simulink library "helperLib"  (R2016a)
settings: Solver=ode45  StartTime=0.0  StopTime=10.0  RelTol=1e-3
values from neighbouring files (symbols this model uses):
  atanDomain = 5    [rev0BB_setup.m]
  atanResolution = 2^-9    (= 0.001953125)    [rev0BB_setup.m]
  averaging_denom = zeros(1, averaging_samples)    [rev0BB_setup.m]
  averaging_num = ones(1, averaging_samples)    [rev0BB_setup.m]
  frac_lut_domain = 256    [rev0BB_setup.m]
  frac_lut_res = 2^-5    (= 0.03125)    [rev0BB_setup.m]
  mult_pipeline = 1    [rev0BB_setup.m]
  regular_pipeline = 1    [rev0BB_setup.m]
libraries: helperLib x11, simulink x8
settings Model: Creator=cyarp  LastModifiedBy=Christopher Yarp
settings DataIOCC: LimitDataPoints=on  SaveFormat=Array
settings DebuggingCC: SolverPrmCheckMsg=warning
settings HardwareCC: ProdBitPerPointer=32  ProdLargestAtomicFloat=None  ProdIntDivRoundTo=Undefined  ProdEndianess=Unspecified  ProdWordSize=32  ProdHWDeviceType=32-bit Generic
settings ModelReferenceCC: PropagateSignalLabelsOutOfModel=off
settings ConfigComp: CovModelRefEnable=Off  CovSFcnEnable=off

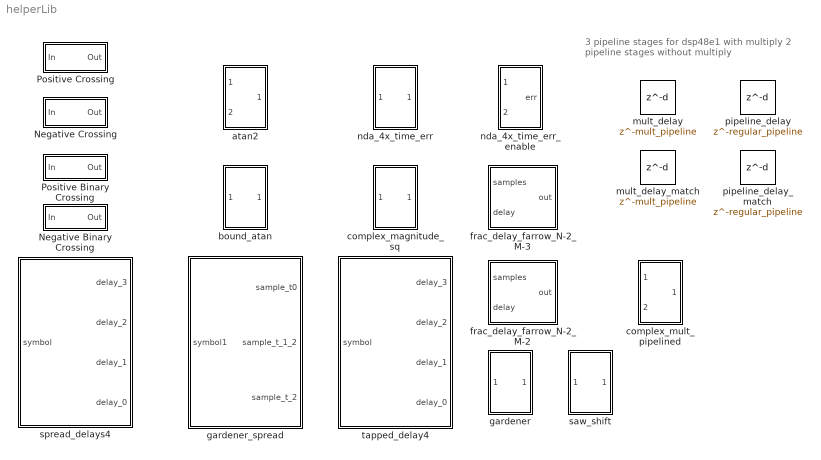
== system helperLib ==
  note: 3 pipeline stages for dsp48e1 with multiply
      | 2 pipeline stages without multiply
  Negative Binary Crossing : Subsystem
  Negative Crossing : Subsystem  mask{crossPt=0}
      mask prompts: crossPt "Crossing Point"
      mask help:
      | Negative Crossing
      | Will output true if goes greater than or equal to threshold to less than
      | theshold.  Will output zero otherwise.
      mask Display: fprintf('-Cross (%d)', crossPt)
  Positive Binary Crossing : Subsystem
  Positive Crossing : Subsystem  mask{crossPt=0}
      mask prompts: crossPt "Crossing Pt"
      mask help:
      | Positive Crossing
      | Will output true if goes from below threshold to greater than or equal to
      | theshold.  Will output zero otherwise.
      mask Display: fprintf('+Cross (%d)', crossPt)
  atan2 : Subsystem
  bound_atan : Subsystem
  complex_magnitude_sq : Subsystem
  complex_mult_pipelined : Subsystem
  frac_delay_farrow_N-2_M-2 : Subsystem
  frac_delay_farrow_N-2_M-3 : Subsystem
  gardener : Subsystem
  gardener_spread : Subsystem
  mult_delay : Delay  DelayLength=mult_pipeline
  mult_delay_match : Delay  DelayLength=mult_pipeline
  nda_4x_time_err : Subsystem
  nda_4x_time_err_enable : Subsystem
  pipeline_delay : Delay  DelayLength=regular_pipeline
  pipeline_delay_match : Delay  DelayLength=regular_pipeline
  saw_shift : Subsystem
  spread_delays4 : Subsystem
  "tapped_delay4 " : Subsystem

== system helperLib/Negative Binary Crossing ==
  In : Inport  OutDataTypeStr=boolean
  Delay : Delay  DelayLength=1  InitialCondition=0
  Logical Operator : Logic  AllPortsSameDT=off  OutDataTypeStr=boolean
  Logical Operator1 : Logic  Operator=NOT  Inputs=1  AllPortsSameDT=off  OutDataTypeStr=boolean
  Out : Outport  OutDataTypeStr=boolean
  wires:
  In/1 -> Logical Operator1/1, Delay/1
  Logical Operator/1 -> Out/1
  Logical Operator1/1 -> Logical Operator/1
  Delay/1 -> Logical Operator/2

== system helperLib/Negative Crossing ==
  In : Inport
  Compare To Constant : simulink/Logic and Bit Operations/Compare To Constant  relop=<  const=crossPt  OutDataTypeStr=boolean
  Compare To Constant1 : simulink/Logic and Bit Operations/Compare To Constant  relop=>=  const=crossPt  OutDataTypeStr=boolean
  Delay : Delay  DelayLength=1  InitialCondition=0
  Logical Operator : Logic  AllPortsSameDT=off  OutDataTypeStr=boolean
  Out : Outport  OutDataTypeStr=boolean
  wires:
  Logical Operator/1 -> Out/1
  In/1 -> Compare To Constant1/1, Compare To Constant/1
  Compare To Constant/1 -> Logical Operator/1
  Compare To Constant1/1 -> Delay/1
  Delay/1 -> Logical Operator/2

== system helperLib/Positive Binary Crossing ==
  In : Inport  OutDataTypeStr=boolean
  Delay : Delay  DelayLength=1  InitialCondition=0
  Logical Operator : Logic  AllPortsSameDT=off  OutDataTypeStr=boolean
  Logical Operator1 : Logic  Operator=NOT  Inputs=1  AllPortsSameDT=off  OutDataTypeStr=boolean
  Out : Outport  OutDataTypeStr=boolean
  wires:
  In/1 -> Logical Operator/1, Delay/1
  Logical Operator/1 -> Out/1
  Delay/1 -> Logical Operator1/1
  Logical Operator1/1 -> Logical Operator/2

== system helperLib/Positive Crossing ==
  In : Inport
  Compare To Constant : simulink/Logic and Bit Operations/Compare To Constant  relop=>=  const=crossPt  OutDataTypeStr=boolean
  Compare To Constant1 : simulink/Logic and Bit Operations/Compare To Constant  relop=<  const=crossPt  OutDataTypeStr=boolean
  Delay : Delay  DelayLength=1  InitialCondition=0
  Logical Operator : Logic  AllPortsSameDT=off  OutDataTypeStr=boolean
  Out : Outport  OutDataTypeStr=boolean
  wires:
  Compare To Constant1/1 -> Delay/1
  Compare To Constant/1 -> Logical Operator/1
  Logical Operator/1 -> Out/1
  In/1 -> Compare To Constant1/1, Compare To Constant/1
  Delay/1 -> Logical Operator/2

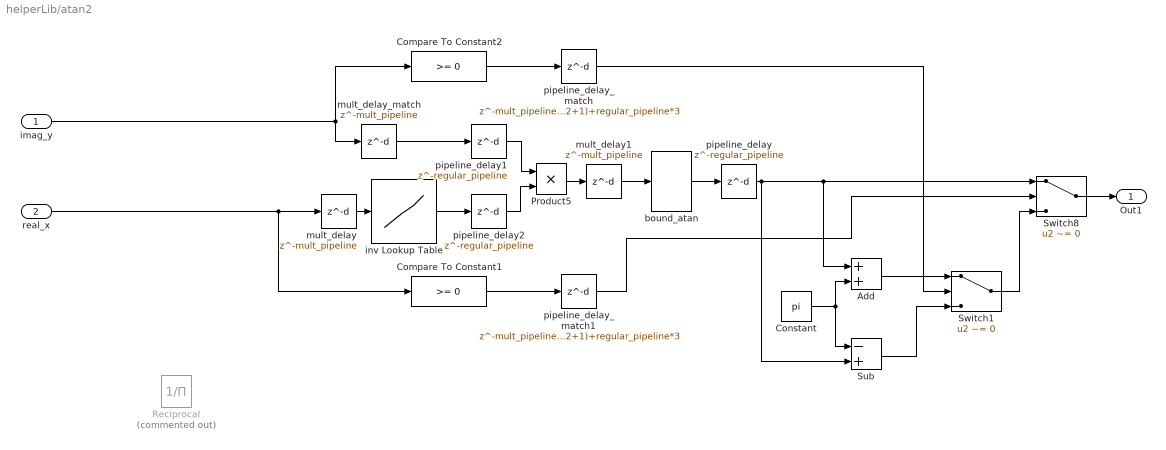
== system helperLib/atan2 ==
  imag_y : Inport
  real_x : Inport  Port=2
  Add : Sum
  Compare To Constant1 : simulink/Logic and Bit Operations/Compare To Constant  relop=>=  const=0  OutDataTypeStr=boolean
  Compare To Constant2 : simulink/Logic and Bit Operations/Compare To Constant  relop=>=  const=0  OutDataTypeStr=boolean
  Constant : Constant  Value=pi  OutDataTypeStr=Inherit: Inherit via back propagation  SampleTime=-1
  Product5 : Product  OutDataTypeStr=Inherit: Same as first input
  Reciprocal : Product  Commented=on  Inputs=/  SaturateOnIntegerOverflow=on  RndMeth=Zero
  Sub : Sum  Inputs=-+
  Switch1 : Switch  Criteria=u2 ~= 0  OutDataTypeStr=Inherit: Inherit via back propagation
  Switch8 : Switch  Criteria=u2 ~= 0  OutDataTypeStr=Inherit: Inherit via back propagation
  bound_atan : helperLib/bound_atan
  inv Lookup Table : Lookup_n-D  NumberOfTableDimensions=1  BreakpointsForDimension1=-frac_lut_domain:frac_lut_res:frac_lut_domain  IndexSearchMethod=Evenly spaced points  Table=ones(size(-frac_lut_domain:frac_lut_res:frac_lut_domain))./(-frac_lut_domain:frac_lut_res:frac_lut_domain)  InterpMethod=Flat  DiagnosticForOutOfRangeInput=Error  InternalRulePriority=Speed  RndMeth=Simplest  InputSameDT=on
  mult_delay : Delay  DelayLength=mult_pipeline
  mult_delay1 : Delay  DelayLength=mult_pipeline
  mult_delay_match : Delay  DelayLength=mult_pipeline
  pipeline_delay : Delay  DelayLength=regular_pipeline
  pipeline_delay1 : Delay  DelayLength=regular_pipeline
  pipeline_delay2 : Delay  DelayLength=regular_pipeline
  pipeline_delay_match : Delay  DelayLength=mult_pipeline*(2+1)+regular_pipeline*3
  pipeline_delay_match1 : Delay  DelayLength=mult_pipeline*(2+1)+regular_pipeline*3
  Out1 : Outport
  wires:
  inv Lookup Table/1 -> pipeline_delay2/1
  Product5/1 -> mult_delay1/1
  bound_atan/1 -> pipeline_delay/1
  mult_delay_match/1 -> pipeline_delay1/1
  pipeline_delay/1 -> Sub/2, Add/1, Switch8/1
  Compare To Constant1/1 -> pipeline_delay_match1/1
  Compare To Constant2/1 -> pipeline_delay_match/1
  Switch1/1 -> Switch8/3
  Add/1 -> Switch1/1
  Constant/1 -> Add/2, Sub/1
  Sub/1 -> Switch1/3
  Switch8/1 -> Out1/1
  imag_y/1 -> mult_delay_match/1, Compare To Constant2/1
  pipeline_delay_match1/1 -> Switch8/2
  pipeline_delay_match/1 -> Switch1/2
  real_x/1 -> mult_delay/1, Compare To Constant1/1
  mult_delay/1 -> inv Lookup Table/1
  pipeline_delay1/1 -> Product5/1
  pipeline_delay2/1 -> Product5/2
  mult_delay1/1 -> bound_atan/1

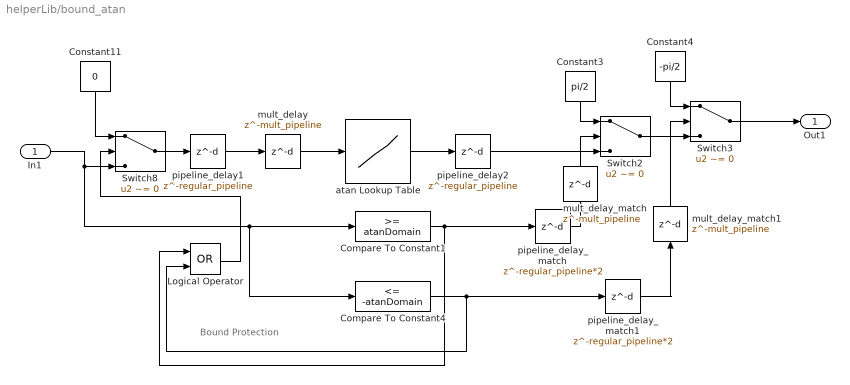
== system helperLib/bound_atan ==
  note: Bound Protection
  In1 : Inport
  Compare To Constant1 : simulink/Logic and Bit Operations/Compare To Constant  relop=>=  const=atanDomain  OutDataTypeStr=boolean
  Compare To Constant4 : simulink/Logic and Bit Operations/Compare To Constant  relop=<=  const=-atanDomain  OutDataTypeStr=boolean
  Constant11 : Constant  Value=0  OutDataTypeStr=Inherit: Inherit via back propagation  SampleTime=-1
  Constant3 : Constant  Value=pi/2  OutDataTypeStr=Inherit: Inherit via back propagation  SampleTime=-1
  Constant4 : Constant  Value=-pi/2  OutDataTypeStr=Inherit: Inherit via back propagation  SampleTime=-1
  Logical Operator : Logic  Operator=OR  AllPortsSameDT=off  OutDataTypeStr=boolean
  Switch2 : Switch  Criteria=u2 ~= 0  OutDataTypeStr=Inherit: Inherit via back propagation
  Switch3 : Switch  Criteria=u2 ~= 0  OutDataTypeStr=Inherit: Inherit via back propagation
  Switch8 : Switch  Criteria=u2 ~= 0  OutDataTypeStr=Inherit: Inherit via back propagation
  atan Lookup Table : Lookup_n-D  NumberOfTableDimensions=1  BreakpointsForDimension1=[-atanDomain:atanResolution:atanDomain]  IndexSearchMethod=Evenly spaced points  Table=atan([-atanDomain:atanResolution:atanDomain])  InterpMethod=Flat  DiagnosticForOutOfRangeInput=Error  RemoveProtectionInput=on  InternalRulePriority=Speed  RndMeth=Simplest  InputSameDT=on
  mult_delay : Delay  DelayLength=mult_pipeline
  mult_delay_match : Delay  DelayLength=mult_pipeline
  mult_delay_match1 : Delay  DelayLength=mult_pipeline
  pipeline_delay1 : Delay  DelayLength=regular_pipeline
  pipeline_delay2 : Delay  DelayLength=regular_pipeline
  pipeline_delay_match : Delay  DelayLength=regular_pipeline*2
  pipeline_delay_match1 : Delay  DelayLength=regular_pipeline*2
  Out1 : Outport
  wires:
  Compare To Constant1/1 -> Logical Operator/1, pipeline_delay_match/1
  Compare To Constant4/1 -> Logical Operator/2, pipeline_delay_match1/1
  Constant3/1 -> Switch2/1
  Switch2/1 -> Switch3/3
  Constant4/1 -> Switch3/1
  Switch3/1 -> Out1/1
  In1/1 -> Switch8/3, Compare To Constant1/1, Compare To Constant4/1
  Logical Operator/1 -> Switch8/2
  Constant11/1 -> Switch8/1
  Switch8/1 -> pipeline_delay1/1
  atan Lookup Table/1 -> pipeline_delay2/1
  pipeline_delay_match/1 -> mult_delay_match/1
  pipeline_delay_match1/1 -> mult_delay_match1/1
  mult_delay_match/1 -> Switch2/2
  mult_delay_match1/1 -> Switch3/2
  pipeline_delay1/1 -> mult_delay/1
  mult_delay/1 -> atan Lookup Table/1
  pipeline_delay2/1 -> Switch2/3

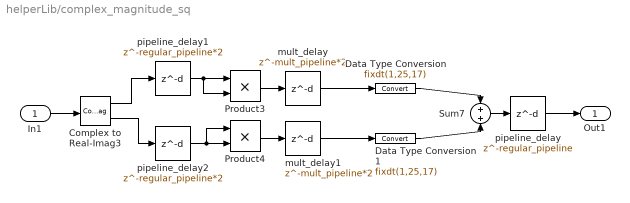
== system helperLib/complex_magnitude_sq ==
  In1 : Inport
  Complex to Real-Imag3 : ComplexToRealImag
  Data Type Conversion : DataTypeConversion  OutDataTypeStr=fixdt(1,25,17)
  Data Type Conversion1 : DataTypeConversion  OutDataTypeStr=fixdt(1,25,17)
  Product3 : Product
  Product4 : Product
  Sum7 : Sum  OutDataTypeStr=Inherit: Same as first input
  mult_delay : Delay  DelayLength=mult_pipeline*2
  mult_delay1 : Delay  DelayLength=mult_pipeline*2
  pipeline_delay : Delay  DelayLength=regular_pipeline
  pipeline_delay1 : Delay  DelayLength=regular_pipeline*2
  pipeline_delay2 : Delay  DelayLength=regular_pipeline*2
  Out1 : Outport
  wires:
  Sum7/1 -> pipeline_delay/1
  Product4/1 -> mult_delay1/1
  Product3/1 -> mult_delay/1
  In1/1 -> Complex to Real-Imag3/1
  Complex to Real-Imag3/1 -> pipeline_delay1/1
  Complex to Real-Imag3/2 -> pipeline_delay2/1
  pipeline_delay1/1 -> Product3/2, Product3/1
  pipeline_delay2/1 -> Product4/1, Product4/2
  mult_delay/1 -> Data Type Conversion/1
  mult_delay1/1 -> Data Type Conversion1/1
  pipeline_delay/1 -> Out1/1
  Data Type Conversion/1 -> Sum7/1
  Data Type Conversion1/1 -> Sum7/2

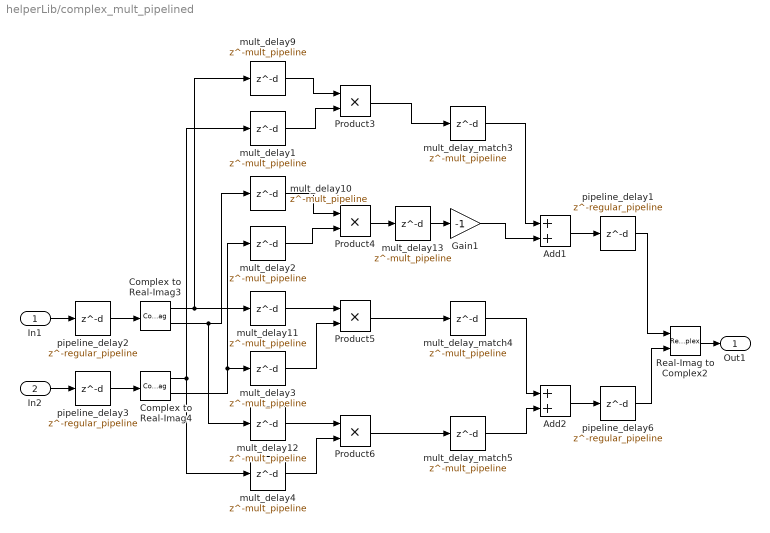
== system helperLib/complex_mult_pipelined ==
  In1 : Inport
  In2 : Inport  Port=2
  Add1 : Sum  OutDataTypeStr=Inherit: Same as first input
  Add2 : Sum  OutDataTypeStr=Inherit: Same as first input
  Complex to Real-Imag3 : ComplexToRealImag
  Complex to Real-Imag4 : ComplexToRealImag
  Gain1 : Gain  Gain=-1  OutDataTypeStr=Inherit: Same as input
  Product{3..6} (4 alike) : Product  OutDataTypeStr=Inherit: Same as first input
  Real-Imag to Complex2 : RealImagToComplex
  mult_delay{1..4,9..13} (9 alike) : Delay  DelayLength=mult_pipeline
  mult_delay_match3 : Delay  DelayLength=mult_pipeline
  mult_delay_match4 : Delay  DelayLength=mult_pipeline
  mult_delay_match5 : Delay  DelayLength=mult_pipeline
  pipeline_delay{1..3,6} (4 alike) : Delay  DelayLength=regular_pipeline
  Out1 : Outport
  wires:
  Product4/1 -> mult_delay13/1
  Product3/1 -> mult_delay_match3/1
  Product6/1 -> mult_delay_match5/1
  mult_delay_match4/1 -> Add2/1
  Complex to Real-Imag3/2 -> mult_delay12/1, mult_delay10/1
  mult_delay_match3/1 -> Add1/1
  Product5/1 -> mult_delay_match4/1
  Complex to Real-Imag4/1 -> mult_delay1/1, mult_delay4/1
  Real-Imag to Complex2/1 -> Out1/1
  pipeline_delay6/1 -> Real-Imag to Complex2/2
  In2/1 -> pipeline_delay3/1
  pipeline_delay1/1 -> Real-Imag to Complex2/1
  Complex to Real-Imag3/1 -> mult_delay9/1, mult_delay11/1
  mult_delay_match5/1 -> Add2/2
  Gain1/1 -> Add1/2
  Complex to Real-Imag4/2 -> mult_delay3/1, mult_delay2/1
  In1/1 -> pipeline_delay2/1
  Add1/1 -> pipeline_delay1/1
  Add2/1 -> pipeline_delay6/1
  pipeline_delay2/1 -> Complex to Real-Imag3/1
  pipeline_delay3/1 -> Complex to Real-Imag4/1
  mult_delay9/1 -> Product3/1
  mult_delay1/1 -> Product3/2
  mult_delay10/1 -> Product4/1
  mult_delay2/1 -> Product4/2
  mult_delay13/1 -> Gain1/1
  mult_delay11/1 -> Product5/1
  mult_delay3/1 -> Product5/2
  mult_delay12/1 -> Product6/1
  mult_delay4/1 -> Product6/2

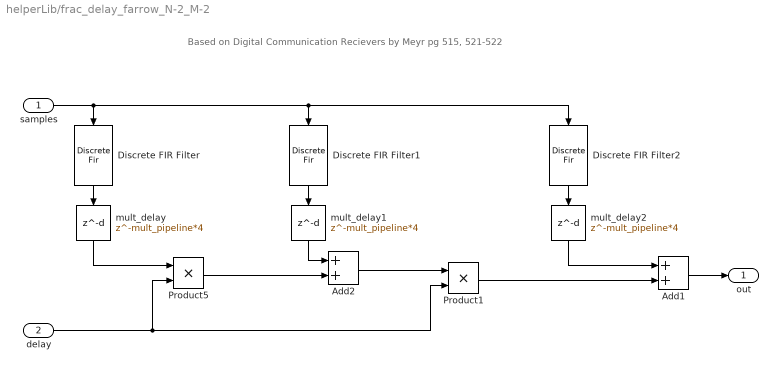
== system helperLib/frac_delay_farrow_N-2_M-2 ==
  note: Based on Digital Communication Recievers by Meyr pg 515, 521-522
  samples : Inport
  delay : Inport  Port=2
  Add1 : Sum  OutDataTypeStr=Inherit: Same as first input
  Add2 : Sum  OutDataTypeStr=Inherit: Same as first input
  Discrete FIR Filter : DiscreteFir  Coefficients=[-0.36881, -0.34303, -0.34303, 0.36881]  OutDataTypeStr=Inherit: Same as input
  Discrete FIR Filter1 : DiscreteFir  Coefficients=[-0.36881, -0.65696, 1.34303, -0.36881]  OutDataTypeStr=Inherit: Same as input
  Discrete FIR Filter2 : DiscreteFir  Coefficients=[0, 1, 0, 0]  OutDataTypeStr=Inherit: Same as input
  Product1 : Product  OutDataTypeStr=Inherit: Same as first input
  Product5 : Product  OutDataTypeStr=Inherit: Same as first input
  mult_delay : Delay  DelayLength=mult_pipeline*4
  mult_delay1 : Delay  DelayLength=mult_pipeline*4
  mult_delay2 : Delay  DelayLength=mult_pipeline*4
  out : Outport
  wires:
  samples/1 -> Discrete FIR Filter2/1, Discrete FIR Filter1/1, Discrete FIR Filter/1
  delay/1 -> Product5/2, Product1/2
  Discrete FIR Filter2/1 -> mult_delay2/1
  Discrete FIR Filter1/1 -> mult_delay1/1
  Add2/1 -> Product1/1
  Discrete FIR Filter/1 -> mult_delay/1
  Add1/1 -> out/1
  mult_delay/1 -> Product5/1
  mult_delay1/1 -> Add2/1
  Product5/1 -> Add2/2
  Product1/1 -> Add1/2
  mult_delay2/1 -> Add1/1

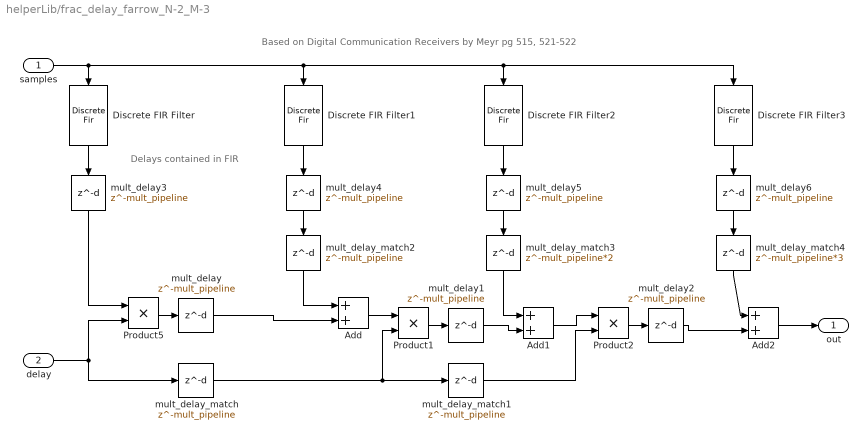
== system helperLib/frac_delay_farrow_N-2_M-3 ==
  note: Delays contained in FIR
  note: Based on Digital Communication Receivers by Meyr pg 515, 521-522
  samples : Inport
  delay : Inport  Port=2
  Add : Sum
  Add1 : Sum
  Add2 : Sum
  Discrete FIR Filter : DiscreteFir  FilterStructure=Direct form transposed  Coefficients=[-0.22485, 0.64567, -0.64567, 0.22485]  OutDataTypeStr=Inherit: Same as input
  Discrete FIR Filter1 : DiscreteFir  FilterStructure=Direct form transposed  Coefficients=[0.70609, -1.31155, 0.62547, 0.03154]  OutDataTypeStr=Inherit: Same as input
  Discrete FIR Filter2 : DiscreteFir  FilterStructure=Direct form transposed  Coefficients=[-0.48124, -0.33413, 1.02020, -0.25639]  OutDataTypeStr=Inherit: Same as input
  Discrete FIR Filter3 : DiscreteFir  FilterStructure=Direct form transposed  Coefficients=[0, 1, 0, 0]  OutDataTypeStr=Inherit: Same as input
  Product1 : Product  OutDataTypeStr=Inherit: Same as first input
  Product2 : Product  OutDataTypeStr=Inherit: Same as first input
  Product5 : Product  OutDataTypeStr=Inherit: Same as first input
  mult_delay{,1..6} (7 alike) : Delay  DelayLength=mult_pipeline
  mult_delay_match : Delay  DelayLength=mult_pipeline
  mult_delay_match1 : Delay  DelayLength=mult_pipeline
  mult_delay_match2 : Delay  DelayLength=mult_pipeline
  mult_delay_match3 : Delay  DelayLength=mult_pipeline*2
  mult_delay_match4 : Delay  DelayLength=mult_pipeline*3
  out : Outport
  wires:
  mult_delay_match4/1 -> Add2/1
  mult_delay_match3/1 -> Add1/1
  mult_delay_match2/1 -> Add/1
  mult_delay_match1/1 -> Product2/2
  mult_delay_match/1 -> mult_delay_match1/1, Product1/2
  mult_delay2/1 -> Add2/2
  mult_delay1/1 -> Add1/2
  Add2/1 -> out/1
  Product2/1 -> mult_delay2/1
  Add1/1 -> Product2/1
  mult_delay5/1 -> mult_delay_match3/1
  Product1/1 -> mult_delay1/1
  Add/1 -> Product1/1
  mult_delay/1 -> Add/2
  mult_delay4/1 -> mult_delay_match2/1
  Discrete FIR Filter3/1 -> mult_delay6/1
  Discrete FIR Filter1/1 -> mult_delay4/1
  Discrete FIR Filter2/1 -> mult_delay5/1
  Discrete FIR Filter/1 -> mult_delay3/1
  samples/1 -> Discrete FIR Filter3/1, Discrete FIR Filter2/1, Discrete FIR Filter1/1, Discrete FIR Filter/1
  Product5/1 -> mult_delay/1
  delay/1 -> mult_delay_match/1, Product5/2
  mult_delay3/1 -> Product5/1
  mult_delay6/1 -> mult_delay_match4/1

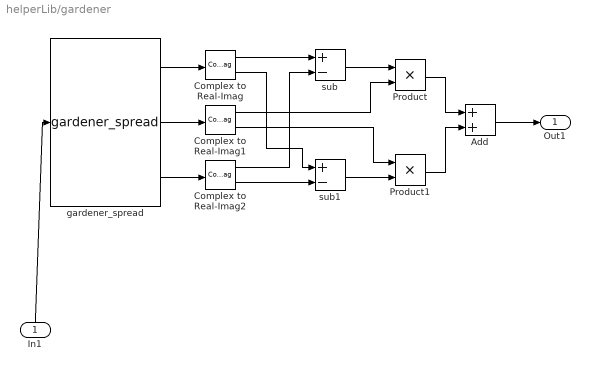
== system helperLib/gardener ==
  In1 : Inport
  Add : Sum
  Complex to Real-Imag : ComplexToRealImag
  Complex to Real-Imag1 : ComplexToRealImag
  Complex to Real-Imag2 : ComplexToRealImag
  Product : Product
  Product1 : Product
  gardener_spread : helperLib/gardener_spread
  sub : Sum  Inputs=+-
  sub1 : Sum  Inputs=+-
  Out1 : Outport
  wires:
  gardener_spread/2 -> Complex to Real-Imag1/1
  gardener_spread/1 -> Complex to Real-Imag/1
  Complex to Real-Imag2/2 -> sub1/2
  gardener_spread/3 -> Complex to Real-Imag2/1
  Complex to Real-Imag2/1 -> sub/2
  Complex to Real-Imag1/2 -> Product1/1
  Add/1 -> Out1/1
  sub1/1 -> Product1/2
  Complex to Real-Imag1/1 -> Product/2
  Complex to Real-Imag/1 -> sub/1
  Product/1 -> Add/1
  Complex to Real-Imag/2 -> sub1/1
  sub/1 -> Product/1
  Product1/1 -> Add/2
  In1/1 -> gardener_spread/1

== system helperLib/gardener_spread ==
  symbol1 : Inport
  Delay : Delay  DelayLength=1  InitialCondition=0
  Downsample3 : DownSample  N=4  RateOptions=Allow multirate processing
  Downsample4 : DownSample  N=4  RateOptions=Allow multirate processing
  Downsample6 : DownSample  N=4  phase=2  RateOptions=Allow multirate processing
  sample_t0 : Outport
  sample_t_1_2 : Outport  Port=2
  sample_t_2 : Outport  Port=3
  wires:
  symbol1/1 -> Delay/1, Downsample4/1, Downsample6/1
  Downsample6/1 -> sample_t_1_2/1
  Downsample4/1 -> sample_t0/1
  Downsample3/1 -> sample_t_2/1
  Delay/1 -> Downsample3/1

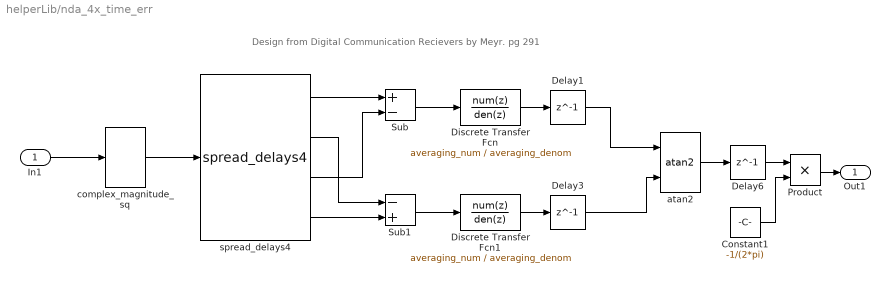
== system helperLib/nda_4x_time_err ==
  note: Design from Digital Communication Recievers by Meyr. pg 291
  In1 : Inport
  Constant1 : Constant  Value=-1/(2*pi)  OutDataTypeStr=Inherit: Inherit via back propagation  SampleTime=-1
  Delay1 : Delay  DelayLength=1  InitialCondition=0
  Delay3 : Delay  DelayLength=1  InitialCondition=0
  Delay6 : Delay  DelayLength=1  InitialCondition=0
  Discrete Transfer Fcn : DiscreteTransferFcn  Numerator=averaging_num  Denominator=averaging_denom  OutDataTypeStr=Inherit: Same as input
  Discrete Transfer Fcn1 : DiscreteTransferFcn  Numerator=averaging_num  Denominator=averaging_denom  OutDataTypeStr=Inherit: Same as input
  Product : Product  OutDataTypeStr=Inherit: Same as first input
  Sub : Sum  Inputs=+-
  Sub1 : Sum  Inputs=-+
  atan2 : helperLib/atan2
  complex_magnitude_sq : helperLib/complex_magnitude_sq
  spread_delays4 : helperLib/spread_delays4
  Out1 : Outport
  wires:
  atan2/1 -> Delay6/1
  Sub1/1 -> Discrete Transfer Fcn1/1
  Constant1/1 -> Product/2
  spread_delays4/4 -> Sub1/2
  spread_delays4/1 -> Sub/1
  Delay6/1 -> Product/1
  Sub/1 -> Discrete Transfer Fcn/1
  complex_magnitude_sq/1 -> spread_delays4/1
  spread_delays4/2 -> Sub1/1
  Discrete Transfer Fcn/1 -> Delay1/1
  Delay1/1 -> atan2/1
  Product/1 -> Out1/1
  spread_delays4/3 -> Sub/2
  In1/1 -> complex_magnitude_sq/1
  Discrete Transfer Fcn1/1 -> Delay3/1
  Delay3/1 -> atan2/2

== system helperLib/nda_4x_time_err_enable ==
  note: Design from Digital Communication Recievers by Meyr. pg 291, 529
  samples : Inport
  enable : Inport  Port=2
  phase_est : Subsystem
  "tapped_delay4 " : helperLib/tapped_delay4 
  err : Outport
  wires:
  samples/1 -> "tapped_delay4 "/1
  enable/1 -> phase_est/Enable
  phase_est/1(Out1) -> err/1
  "tapped_delay4 "/2 -> phase_est/2(In2)
  "tapped_delay4 "/1 -> phase_est/1(In1)
  "tapped_delay4 "/4 -> phase_est/4(In4)
  "tapped_delay4 "/3 -> phase_est/3(In3)

== system helperLib/saw_shift ==
  In1 : Inport
  Constant3 : Constant  Value=0.5  OutDataTypeStr=Inherit: Inherit via back propagation  SampleTime=-1
  Data Type Conversion : DataTypeConversion  OutDataTypeStr=int8
  Data Type Conversion1 : DataTypeConversion
  Sub : Sum  Inputs=+-
  Sub1 : Sum  Inputs=+-
  Sub2 : Sum  Inputs=+-
  Out1 : Outport
  wires:
  Sub1/1 -> Sub2/1
  Constant3/1 -> Sub2/2, Sub/2
  Sub/1 -> Sub1/1, Data Type Conversion/1
  Data Type Conversion1/1 -> Sub1/2
  In1/1 -> Sub/1
  Data Type Conversion/1 -> Data Type Conversion1/1
  Sub2/1 -> Out1/1

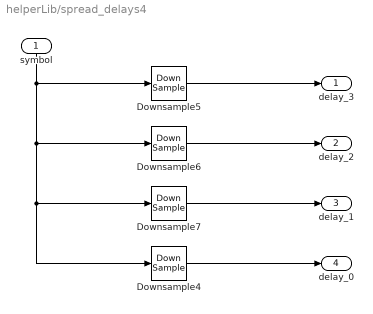
== system helperLib/spread_delays4 ==
  symbol : Inport
  Downsample4 : DownSample  N=4  RateOptions=Allow multirate processing
  Downsample5 : DownSample  N=4  phase=3  RateOptions=Allow multirate processing
  Downsample6 : DownSample  N=4  phase=2  RateOptions=Allow multirate processing
  Downsample7 : DownSample  N=4  phase=1  RateOptions=Allow multirate processing
  delay_3 : Outport
  delay_2 : Outport  Port=2
  delay_1 : Outport  Port=3
  delay_0 : Outport  Port=4
  wires:
  symbol/1 -> Downsample4/1, Downsample7/1, Downsample6/1, Downsample5/1
  Downsample5/1 -> delay_3/1
  Downsample6/1 -> delay_2/1
  Downsample7/1 -> delay_1/1
  Downsample4/1 -> delay_0/1

== system helperLib/tapped_delay4  ==
  symbol : Inport
  Delay : Delay  DelayLength=1  InitialCondition=0
  Delay1 : Delay  DelayLength=1  InitialCondition=0
  Delay2 : Delay  DelayLength=1  InitialCondition=0
  delay_3 : Outport
  delay_2 : Outport  Port=2
  delay_1 : Outport  Port=3
  delay_0 : Outport  Port=4
  wires:
  symbol/1 -> Delay/1, delay_0/1
  Delay/1 -> Delay1/1, delay_1/1
  Delay1/1 -> Delay2/1, delay_2/1
  Delay2/1 -> delay_3/1

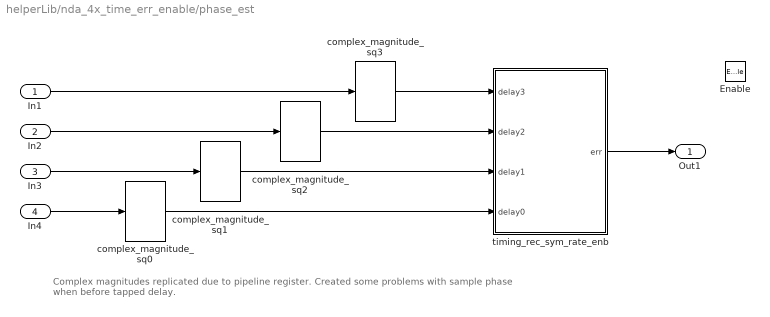
== system helperLib/nda_4x_time_err_enable/phase_est ==
  note: Complex magnitudes replicated due to pipeline register. Created some problems with sample phase when before tapped delay.
  In1 : Inport
  In2 : Inport  Port=2
  In3 : Inport  Port=3
  In4 : Inport  Port=4
  Enable : EnablePort
  complex_magnitude_sq{0..3} (4 alike) : helperLib/complex_magnitude_sq
  timing_rec_sym_rate_enb : Subsystem
  Out1 : Outport  InitialOutput=[0]
  wires:
  timing_rec_sym_rate_enb/1(err) -> Out1/1
  complex_magnitude_sq0/1 -> timing_rec_sym_rate_enb/4(delay0)
  complex_magnitude_sq3/1 -> timing_rec_sym_rate_enb/1(delay3)
  complex_magnitude_sq2/1 -> timing_rec_sym_rate_enb/2(delay2)
  complex_magnitude_sq1/1 -> timing_rec_sym_rate_enb/3(delay1)
  In1/1 -> complex_magnitude_sq3/1
  In4/1 -> complex_magnitude_sq0/1
  In3/1 -> complex_magnitude_sq1/1
  In2/1 -> complex_magnitude_sq2/1

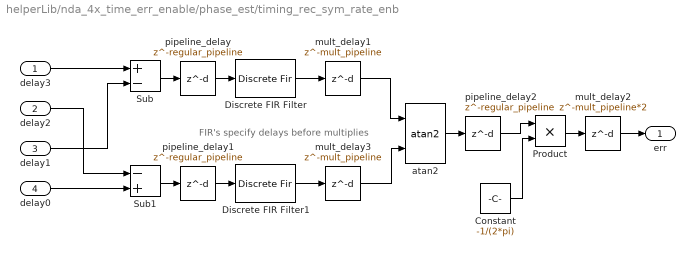
== system helperLib/nda_4x_time_err_enable/phase_est/timing_rec_sym_rate_enb ==
  note: FIR's specify delays before multiplies
  delay3 : Inport
  delay2 : Inport  Port=2
  delay1 : Inport  Port=3
  delay0 : Inport  Port=4
  Constant : Constant  Value=-1/(2*pi)  OutDataTypeStr=Inherit: Inherit via back propagation  SampleTime=-1
  Discrete FIR Filter : DiscreteFir  FilterStructure=Direct form symmetric  Coefficients=averaging_num  OutDataTypeStr=Inherit: Same as input
  Discrete FIR Filter1 : DiscreteFir  FilterStructure=Direct form symmetric  Coefficients=averaging_num  OutDataTypeStr=Inherit: Same as input
  Product : Product  OutDataTypeStr=Inherit: Same as first input
  Sub : Sum  Inputs=+-
  Sub1 : Sum  Inputs=-+
  atan2 : helperLib/atan2
  mult_delay1 : Delay  DelayLength=mult_pipeline
  mult_delay2 : Delay  DelayLength=mult_pipeline*2
  mult_delay3 : Delay  DelayLength=mult_pipeline
  pipeline_delay : Delay  DelayLength=regular_pipeline
  pipeline_delay1 : Delay  DelayLength=regular_pipeline
  pipeline_delay2 : Delay  DelayLength=regular_pipeline
  err : Outport
  wires:
  mult_delay3/1 -> atan2/2
  Sub/1 -> pipeline_delay/1
  Discrete FIR Filter/1 -> mult_delay1/1
  delay2/1 -> Sub1/1
  Product/1 -> mult_delay2/1
  mult_delay1/1 -> atan2/1
  delay1/1 -> Sub/2
  Discrete FIR Filter1/1 -> mult_delay3/1
  atan2/1 -> pipeline_delay2/1
  Sub1/1 -> pipeline_delay1/1
  delay0/1 -> Sub1/2
  delay3/1 -> Sub/1
  pipeline_delay/1 -> Discrete FIR Filter/1
  pipeline_delay1/1 -> Discrete FIR Filter1/1
  mult_delay2/1 -> err/1
  pipeline_delay2/1 -> Product/1
  Constant/1 -> Product/2
